simulink model "CC_M8"  (R2017b)
settings: Solver=VariableStepAuto  StartTime=0.0  StopTime=10.0  RelTol=1e-3
undefined symbols (not defined in the file): DiscIntNeverNeededParam, Kdec, KInc, Kp, Kp1

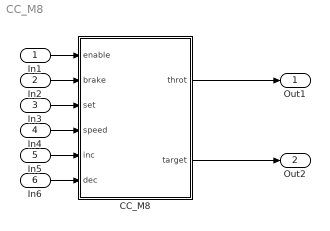
== system CC_M8 ==
  In1 : Inport
  In2 : Inport  Port=2
  In3 : Inport  Port=3
  In4 : Inport  Port=4
  In5 : Inport  Port=5
  In6 : Inport  Port=6
  CC_M8 : Subsystem
  Out1 : Outport
  Out2 : Outport  Port=2
  wires:
  CC_M8/1(throt) -> Out1/1
  In5/1 -> CC_M8/5(inc)
  In1/1 -> CC_M8/1(enable)
  In4/1 -> CC_M8/4(speed)
  CC_M8/2(target) -> Out2/1
  In3/1 -> CC_M8/3(set)
  In2/1 -> CC_M8/2(brake)
  In6/1 -> CC_M8/6(dec)

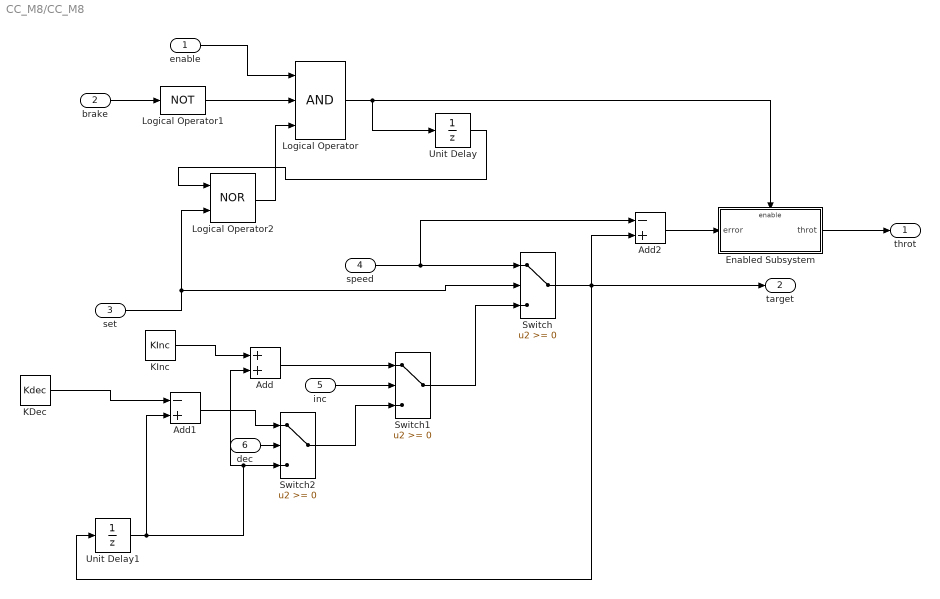
== system CC_M8/CC_M8 ==
  enable : Inport
  brake : Inport  Port=2
  set : Inport  Port=3
  speed : Inport  Port=4
  inc : Inport  Port=5
  dec : Inport  Port=6
  Add : Sum
  Add1 : Sum  Inputs=-+
  Add2 : Sum  Inputs=-+
  Enabled Subsystem : Subsystem  TreatAsAtomicUnit=on
  KDec : Constant  Value=Kdec
  KInc : Constant  Value=KInc
  Logical Operator : Logic  Inputs=3  AllPortsSameDT=off  OutDataTypeStr=boolean
  Logical Operator1 : Logic  Operator=NOT  Inputs=3  AllPortsSameDT=off  OutDataTypeStr=boolean
  Logical Operator2 : Logic  Operator=NOR  AllPortsSameDT=off  OutDataTypeStr=boolean
  Switch : Switch
  Switch1 : Switch
  Switch2 : Switch
  Unit Delay : UnitDelay  InitialCondition=1  SampleTime=-1
  Unit Delay1 : UnitDelay  SampleTime=-1
  throt : Outport
  target : Outport  Port=2
  wires:
  enable/1 -> Logical Operator/1
  Logical Operator1/1 -> Logical Operator/2
  brake/1 -> Logical Operator1/1
  set/1 -> Logical Operator2/2, Switch/2
  Logical Operator/1 -> Enabled Subsystem/Enable, Unit Delay/1
  Unit Delay/1 -> Logical Operator2/1
  Logical Operator2/1 -> Logical Operator/3
  speed/1 -> Add2/1, Switch/1
  Switch1/1 -> Switch/3
  Switch2/1 -> Switch1/3
  Add/1 -> Switch1/1
  inc/1 -> Switch1/2
  dec/1 -> Switch2/2
  Switch/1 -> target/1, Add2/2, Unit Delay1/1
  Unit Delay1/1 -> Add1/2, Add/2, Switch2/3
  KInc/1 -> Add/1
  Add1/1 -> Switch2/1
  KDec/1 -> Add1/1
  Add2/1 -> Enabled Subsystem/1(error)
  Enabled Subsystem/1(throt) -> throt/1

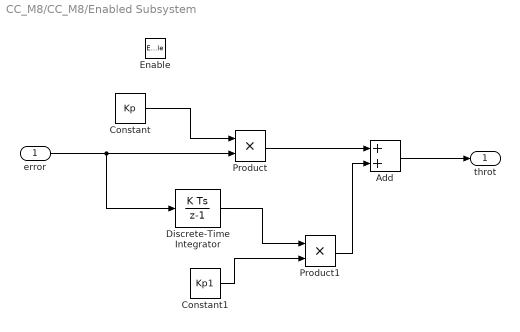
== system CC_M8/CC_M8/Enabled Subsystem ==
  error : Inport
  Enable : EnablePort
  Add : Sum
  Constant : Constant  Value=Kp
  Constant1 : Constant  Value=Kp1
  Discrete-Time Integrator : DiscreteIntegrator  gainval=Ki  ICPrevOutput=DiscIntNeverNeededParam  ICPrevScaledInput=DiscIntNeverNeededParam
  Product : Product
  Product1 : Product
  throt : Outport
  wires:
  Constant/1 -> Product/1
  Product/1 -> Add/1
  Add/1 -> throt/1
  Constant1/1 -> Product1/2
  Product1/1 -> Add/2
  Discrete-Time Integrator/1 -> Product1/1
  error/1 -> Discrete-Time Integrator/1, Product/2
